simulink model "ModelRitm"  (Simulink 9.2)
settings: Solver=ode45  StartTime=0.0  StopTime=1  FixedStep=1/fd/10  MaxStep=100e-6  RelTol=1e-6  EnableMultiTasking=on
libraries: fl_lib x8, nesl_utility x4, pe_lib x1, SimscapeCustomBlocks_lib x1
Description:
  | Copyright 2008-2010 The MathWorks, Inc.
settings Model: Creator=MathWorks  LastModifiedBy=evgeniy.selkov  ExtModeTrigMode=oneshot  ExtModeArmWhenConnect=off  ExtModeAutoUpdateStatusClock=off
settings DataIOCC: LimitDataPoints=off  SignalLoggingName=sigsOut
settings OptimizationCC: BlockReduction=off  BooleanDataType=off  ExpressionDepthLimit=2147483647  InitFltsAndDblsToZero=on  EfficientMapNaN2IntZero=off
settings DebuggingCC: SaveWithParameterizedLinksMsg=none  CheckExecutionContextPreStartOutputMsg=on  CheckExecutionContextRuntimeOutputMsg=on  SignalResolutionControl=TryResolveAllWithWarning  MultiTaskDSMMsg=warning  MultiTaskCondExecSysMsg=none  SigSpecEnsureSampleTimeMsg=none  UnconnectedInputMsg=none  UnconnectedOutputMsg=none  UnconnectedLineMsg=none
settings HardwareCC: ProdHWDeviceType=Specified  TargetUnknown=on
settings GRTTargetCC: TargetFcnLib=ansi_tfl_tmw.mat

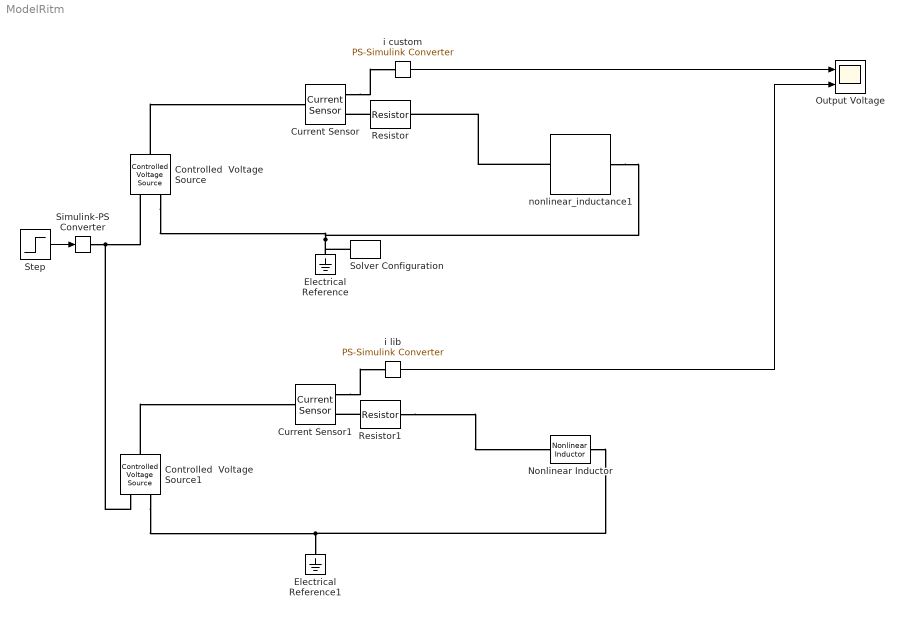
== system ModelRitm ==
  Controlled  Voltage Source : fl_lib/Electrical/Electrical Sources/Controlled Voltage Source
  Controlled  Voltage Source1 : fl_lib/Electrical/Electrical Sources/Controlled Voltage Source
  Current Sensor : fl_lib/Electrical/Electrical Sensors/Current Sensor
  Current Sensor1 : fl_lib/Electrical/Electrical Sensors/Current Sensor
  Electrical Reference : fl_lib/Electrical/Electrical Elements/Electrical Reference
  Electrical Reference1 : fl_lib/Electrical/Electrical Elements/Electrical Reference
  Nonlinear Inductor : pe_lib/Passive Devices/Fundamental Components/Nonlinear Inductor  parameterization_option=3  Nw=20000  L=2e-4 H  L_sat=1e-4 H  current_data=[0, .64, 1.28, 1.92, 2.56, 3.2] A  magnetic_flux_data=[0, 1.29, 2, 2.27, 2.36, 2.39] .* 1e-5 Wb  H_data=[0, 200, 400, 600, 800, 1000] A/m  B_data=[0, .81, 1.25, 1.42, 1.48, 1.49] T  magnetic_flux_sat=1.3e-05 Wb  length_effective=0.032 m  area_effective=1.6e-5 m^2  dBdH0=0.005 m*T/A  B1=1.49 T  H1=1000 A/m  c=0.1  K=200 A/m  alpha=1e-4  x0_option=1  i_L0=0 A  phi0=0 Wb  B0=0 T  H0=0 A/m  averaging_period=0 s  G_parasitic=1e-9 1/Ohm  interpolation_option=1
      settings: SourceProductName=Simscape Power Systems  SourceProductBaseCode=PS
  Output Voltage : Scope  NumInputPorts=2
  Resistor : fl_lib/Electrical/Electrical Elements/Resistor  R=1 Ohm  i_specify=off  i_priority=None  i=0 A  i_nominal_specify=off  i_nominal_unit=A  i_nominal_value=1  v_specify=off  v_priority=None  v=0 V  v_nominal_specify=off  v_nominal_unit=V  v_nominal_value=1
  Resistor1 : fl_lib/Electrical/Electrical Elements/Resistor  R=1 Ohm  i_specify=off  i_priority=None  i=0 A  i_nominal_specify=off  i_nominal_unit=A  i_nominal_value=1  v_specify=off  v_priority=None  v=0 V  v_nominal_specify=off  v_nominal_unit=V  v_nominal_value=1
  Simulink-PS Converter : nesl_utility/Simulink-PS Converter  PhysicalDomain=network_engine_domain  SubClassName=ps_input  LeftPortType=input  RightPortType=output  PseudoPeriodic=off  Frequencies=[]  NoiseDistribution=none  NoiseParameters=[]  Unit=1  AffineConversion=off  FilteringAndDerivatives=provide  SimscapeFilterOrder=1  InputFilterTimeConstant=0.001  UdotUserProvided=0
  Solver Configuration : nesl_utility/Solver Configuration  PhysicalDomain=network_engine_domain  SubClassName=solver  LeftPortType=input  RightPortType=generic  Tones=[]  Harmonics=[]  SimulateNoise=off  Profile=off  UseLocalSampling=off  EnableSwitchedLinearOptims=on  FrequencyDomain=off  UseCCode=off  RelTol=0.001  AbsTol=1e-06  MinStep=1e-09  ToWorkspace=off  RevertToSquareIcSolve=off  NumHomotopyIterations=100  PhasorMode=off  PhasorModeNumHarmonics=1  DoDC=off  ResidualTolerance=1e-6  UseLocalSolver=on  LocalSolverChoice=NE_BACKWARD_EULER_ADVANCER  LocalSolverSampleTime=.001  DoFixedCost=on  MaxNonlinIter=3  MaxModeIter=2  LinearAlgebra=auto  EquationFormulation=NE_TIME_EF  DelaysMemoryBudget=2048  AutomaticFiltering=on  FilteringTimeConstant=0.001  PartitionStorageMethod=AS_NEEDED  PartitionMemoryBudget=1024
  Step : Step  Time=0.2  After=5  SampleTime=0
  i custom : nesl_utility/PS-Simulink Converter  PhysicalDomain=network_engine_domain  SubClassName=ps_output  LeftPortType=input  RightPortType=output  PseudoPeriodic=off  Frequencies=[]  Unit=1  AffineConversion=off
  i lib : nesl_utility/PS-Simulink Converter  PhysicalDomain=network_engine_domain  SubClassName=ps_output  LeftPortType=input  RightPortType=output  PseudoPeriodic=off  Frequencies=[]  Unit=1  AffineConversion=off
  nonlinear_inductance1 : SimscapeCustomBlocks_lib/Electrical/nonlinear_inductance  Nturns=20000  i_vector=[0, .64, 1.28, 1.92, 2.56, 3.2] A  phi_vector=[0, 1.29, 2, 2.27, 2.36, 2.39] * 1e-5 Wb  i_specify=off  i_priority=None  i=0 A  i_nominal_specify=off  i_nominal_unit=A  i_nominal_value=1  v_specify=off  v_priority=None  v=0 V  v_nominal_specify=off  v_nominal_unit=V  v_nominal_value=1  i_L_specify=off  i_L_priority=High  i_L=0 A  i_L_nominal_specify=off  i_L_nominal_unit=A  i_L_nominal_value=1
  wires:
  i custom/1 -> Output Voltage/1
  Step/1 -> Simulink-PS Converter/1
  i lib/1 -> Output Voltage/2
  connections:
  Resistor/LConn1 -- Current Sensor/RConn2
  Current Sensor/RConn1 -- i custom/LConn1
  Simulink-PS Converter/RConn1 -- Controlled  Voltage Source1/RConn1 -- Controlled  Voltage Source/RConn1
  Electrical Reference/LConn1 -- nonlinear_inductance1/RConn1 -- Controlled  Voltage Source/RConn2 -- Solver Configuration/RConn1
  Controlled  Voltage Source/LConn1 -- Current Sensor/LConn1
  nonlinear_inductance1/LConn1 -- Resistor/RConn1
  Controlled  Voltage Source1/RConn2 -- Nonlinear Inductor/RConn1 -- Electrical Reference1/LConn1
  Current Sensor1/RConn1 -- i lib/LConn1
  Controlled  Voltage Source1/LConn1 -- Current Sensor1/LConn1
  Resistor1/LConn1 -- Current Sensor1/RConn2
  Resistor1/RConn1 -- Nonlinear Inductor/LConn1
